simulink model "TCMSSystem"  (R2019b)
settings: configuration reference "ConfigSet_TCMSSystem_Reference" (kept outside this file)
model workspace (MAT data in the model file):
  Prm_TCMSSystem : Simulink.Parameter (value not decoded)
  SampleTime = 0.05
symbols that are objects in the model workspace (value not decoded): Prm_TCMSSystem
undefined symbols (not defined in the file): ADDIntervention, AK1Status, AK2Status, AKContactorStatus, AllDoorsClosed, AllLeftDoorsClosed, AllRightDoorsClosed, APS1Fault, APS1Isolated, APS1OutputVoltage, APS1Status, APS2Fault, APS2Isolated, APS2OutputVoltage, APS2Status, APSKAKContactor, ASCOEnd1, ASCOEnd2, ATBMode, ATCBypassMode, ATCStatusNotOK, ATOMode, ATPLowSpeedCutoutStatus, ATPMode, AuxCompressor, BatteryCurrent, BatteryIsolationContactor, BatteryTemperature, BatteryVoltage, BCG1Fault, BCG1Isolated, BCG1IsolationFailed, BCG1OutputCurrent, BCG1Status, BCG2Fault, BCG2Isolated, BCG2OutputCurrent, BCG2Status, BCGOutputVoltage, BECU1AxleLockedWheelSet1, BECU2AxleLockedWheelSet2, BECUFaulty, BECUMajorFault, BECUMinorFault, BECUStatus, BIC1Inside, BIC1Outside, BIC2Inside, BIC2Outside, Bogie, Bogie1WSPStatus, Bogie2WSPStatus, BogieFaulty, BogieIsolationStatus, BogieSupportedMass, BrakeCylinderPressureGauge, BrakeLoopCBTripped, BrakeLoopOpenTL, BrakeTrainLineStatus, BrakingDemand ... (+215)
libraries: TimersLib x257, simulink x137, LatchesLib x42, VectorOperationsLib x15, TestBenchLib x12, MathOperationsLib x2, FiltersLib x1
(part 6 of 16)

== system TCMSSystem/TCMSSystemPerVehicle/EnabledTCMSVehicle/TCMSElectrical/ElectricalDisplay/FireDetectionScreen ==
  note: FireDetectionScreen
  note: 1. RCCB Tripped
      | 2. Supply Fan Tripped
      | 3. External Smoke Detected
      | 4. Emergency Inverter Tripped
      | 5. HVAC Fire Mode
      | 6. HVAC Reduced Mode
      | 7. HVAC Group MCB Tripped
      | 8. HVAC Major Fault
  BusIn : Inport
  CommonConfig : Inport  Port=2
  In Bus Element : Inport  Port=3  PortName=ElectricalSignals  Element=HVACFaults
  In Bus Element1 : Inport  Port=3  PortName=ElectricalSignals  Element=FDUFailure
  In Bus Element3 : Inport  Port=3  PortName=ElectricalSignals  Element=SmokeAlarmCABArea
  In Bus Element4 : Inport  Port=3  PortName=ElectricalSignals  Element=HeatAlarmEDB
  In Bus Element5 : Inport  Port=3  PortName=ElectricalSignals  Element=FDUStatus
  In Bus Element6 : Inport  Port=3  PortName=ElectricalSignals  Element=SFARStatus
  In Bus Element7 : Inport  Port=3  PortName=ElectricalSignals  Element=UFARStatus
  In Bus Element2 : Inport  Port=3  PortName=ElectricalSignals  Element=InternalFireAlarmTLActive
  In Bus Element9 : Inport  Port=3  PortName=ElectricalSignals  Element=CabActive
  Bus Assignment9 : BusAssignment  AssignedSignals=UnderframeFireAlarmStatus,SaloonFireAlarmStatus,SensorFireAlarmStatus,FireDetectionUnit,InternalFire,ExternalSmoke,SmokeAlarmCABArea,HeatAlarmEDB,FDUFault,SFARFault
  Bus Selector : BusSelector  OutputSignals=HasCab
  Constant : Constant  Value=3
  Constant1 : Constant
  Data Type Conversion{,1..7} (8 alike) : DataTypeConversion
  ExternalSmoke : Selector  InputPortWidth=7  IndexOptions=Index vector (dialog)  Indices=[3]  OutputSizes=1
  FireMode : Selector  InputPortWidth=7  IndexOptions=Index vector (dialog)  Indices=[5]  OutputSizes=1
  OR : Logic  Operator=OR  Inputs=3  AllPortsSameDT=off  OutDataTypeStr=boolean
  OR1 : Logic  AllPortsSameDT=off  OutDataTypeStr=boolean
  OR2 : Logic  AllPortsSameDT=off  OutDataTypeStr=boolean
  OR3 : Logic  Operator=OR  AllPortsSameDT=off  OutDataTypeStr=boolean
  Switch : Switch  Criteria=u2 > Threshold
  BusOut : Outport
  wires:
  BusIn/1 -> Bus Assignment9/1
  Switch/1 -> Bus Assignment9/4
  Bus Assignment9/1 -> BusOut/1
  ExternalSmoke/1 -> Bus Assignment9/7
  In Bus Element/1 -> ExternalSmoke/1, FireMode/1
  OR/1 -> OR1/1, Switch/2
  In Bus Element6/1 -> Data Type Conversion3/1
  In Bus Element3/1 -> Data Type Conversion1/1
  Data Type Conversion/1 -> Bus Assignment9/9
  Data Type Conversion1/1 -> Bus Assignment9/8
  Data Type Conversion2/1 -> Bus Assignment9/5
  Data Type Conversion3/1 -> Bus Assignment9/3
  In Bus Element5/1 -> Data Type Conversion2/1
  In Bus Element1/1 -> OR2/1
  Data Type Conversion4/1 -> Bus Assignment9/10
  In Bus Element7/1 -> Data Type Conversion6/1
  In Bus Element4/1 -> OR3/1, OR/2, Data Type Conversion/1
  Data Type Conversion6/1 -> Bus Assignment9/2
  FireMode/1 -> OR/3
  In Bus Element2/1 -> OR3/2, OR/1
  In Bus Element9/1 -> OR2/2
  OR2/1 -> Data Type Conversion4/1
  Constant/1 -> Switch/1
  Constant1/1 -> Switch/3
  Data Type Conversion5/1 -> Bus Assignment9/6
  Bus Selector/1 -> OR1/2  "<HasCab>"
  OR1/1 -> Data Type Conversion5/1
  CommonConfig/1 -> Bus Selector/1
  OR3/1 -> Data Type Conversion7/1
  Data Type Conversion7/1 -> Bus Assignment9/11

== system TCMSSystem/TCMSSystemPerVehicle/EnabledTCMSVehicle/TCMSElectrical/ElectricalDisplay/FireDetectorScreen ==
  note: MiscellaneaScreen
  BusIn : Inport
  In Bus Element2 : Inport  Port=2  PortName=ElectricalSignals  Element=HeatAlarmEDB
  In Bus Element3 : Inport  Port=2  PortName=ElectricalSignals  Element=SmokeAlarmCABArea
  Bus Assignment7 : BusAssignment  AssignedSignals=HVAC1FireSmokeActive,EDBHeatAlarmActive,CABSmokeAlarmActive
  Bus Selector : BusSelector  OutputSignals=HVACFireMode
  Data Type Conversion : DataTypeConversion
  Data Type Conversion1 : DataTypeConversion
  Data Type Conversion2 : DataTypeConversion
  BusOut : Outport
  wires:
  In Bus Element2/1 -> Data Type Conversion1/1
  Bus Assignment7/1 -> BusOut/1
  BusIn/1 -> Bus Assignment7/1, Bus Selector/1
  Bus Selector/1 -> Data Type Conversion/1  "<HVACFireMode>"
  In Bus Element3/1 -> Data Type Conversion2/1
  Data Type Conversion/1 -> Bus Assignment7/2
  Data Type Conversion1/1 -> Bus Assignment7/3
  Data Type Conversion2/1 -> Bus Assignment7/4

== system TCMSSystem/TCMSSystemPerVehicle/EnabledTCMSVehicle/TCMSElectrical/ElectricalDisplay/HVACScreen ==
  note: HVACScreen
  BusIn : Inport
  In Bus Element : Inport  Port=2  PortName=ElectricalSignals  Element=HVAC1Status
  In Bus Element1 : Inport  Port=2  PortName=ElectricalSignals  Element=HVAC1SetPointTemperature
  In Bus Element2 : Inport  Port=2  PortName=ElectricalSignals  Element=HVAC1IntTemperature
  In Bus Element3 : Inport  Port=2  PortName=ElectricalSignals  Element=HVAC1ExtTemperature
  In Bus Element4 : Inport  Port=2  PortName=ElectricalSignals  Element=HVAC1Faulty
  In Bus Element5 : Inport  Port=2  PortName=ElectricalSignals  Element=HVAC1Isolated
  In Bus Element6 : Inport  Port=2  PortName=ElectricalSignals  Element=HVAC2Status
  In Bus Element7 : Inport  Port=2  PortName=ElectricalSignals  Element=HVAC2SetPointTemperature
  In Bus Element8 : Inport  Port=2  PortName=ElectricalSignals  Element=HVAC2IntTemperature
  In Bus Element9 : Inport  Port=2  PortName=ElectricalSignals  Element=HVAC2ExtTemperature
  In Bus Element10 : Inport  Port=2  PortName=ElectricalSignals  Element=HVAC2Faulty
  In Bus Element11 : Inport  Port=2  PortName=ElectricalSignals  Element=HVAC2Isolated
  In Bus Element12 : Inport  Port=2  PortName=ElectricalSignals  Element=HVACFaults
  In Bus Element13 : Inport  Port=2  PortName=ElectricalSignals  Element=MCBHVACGroupTripped
  In Bus Element16 : Inport  Port=2  PortName=ElectricalSignals  Element=NoOfAPSFailed
  In Bus Element14 : Inport  Port=3  PortName=VehicleFaults  Element=HVAC1ReducedMode
  Bus Assignment1 : BusAssignment  AssignedSignals=HVAC1Status,HVAC1SetPointTemperature,HVAC1InternalTemperature,HVAC1ExternalTemperature,HVAC1Fault,HVAC1Isolated,HVAC2Status,HVAC2SetPointTemperature,HVAC2InternalTemperature,HVAC2ExternalTemperature,HVAC2Fault,HVAC2Isolated,RCCBTripped,SupplyFanTripped,ExtSmokeDetectedinHVAC,EmergencyInverterTripped,HVACFireMode,HVACReducedMode,HVACMajorFault,HVACGroupMCBTripped,HVAC1ReducedMode,HVAC2ReducedMode
  Compare To Constant : simulink/Logic and Bit Operations/Compare To Constant  relop=>=  const=2  OutDataTypeStr=boolean
  Data Type Conversion{1..3,35..38} (7 alike) : DataTypeConversion
  Demux : Demux  Outputs=7
  Logical Operator : Logic  Operator=OR  AllPortsSameDT=off  OutDataTypeStr=boolean
  BusOut : Outport
  wires:
  Data Type Conversion38/1 -> Bus Assignment1/12
  Data Type Conversion37/1 -> Bus Assignment1/13
  In Bus Element3/1 -> Bus Assignment1/5
  In Bus Element8/1 -> Bus Assignment1/10
  In Bus Element1/1 -> Bus Assignment1/3
  Data Type Conversion36/1 -> Bus Assignment1/7
  In Bus Element6/1 -> Bus Assignment1/8
  Data Type Conversion35/1 -> Bus Assignment1/6
  Bus Assignment1/1 -> BusOut/1
  In Bus Element5/1 -> Data Type Conversion36/1
  In Bus Element2/1 -> Bus Assignment1/4
  BusIn/1 -> Bus Assignment1/1
  In Bus Element7/1 -> Bus Assignment1/9
  In Bus Element11/1 -> Data Type Conversion37/1
  In Bus Element10/1 -> Data Type Conversion38/1
  In Bus Element4/1 -> Data Type Conversion35/1
  In Bus Element9/1 -> Bus Assignment1/11
  In Bus Element/1 -> Bus Assignment1/2
  Demux/1 -> Bus Assignment1/14
  Demux/2 -> Bus Assignment1/15
  Demux/3 -> Bus Assignment1/16
  Demux/4 -> Bus Assignment1/17
  Demux/5 -> Bus Assignment1/18
  Demux/6 -> Bus Assignment1/19
  Demux/7 -> Bus Assignment1/20
  In Bus Element12/1 -> Demux/1
  In Bus Element13/1 -> Data Type Conversion1/1
  Data Type Conversion1/1 -> Bus Assignment1/21
  Data Type Conversion2/1 -> Bus Assignment1/22
  Data Type Conversion3/1 -> Bus Assignment1/23
  Compare To Constant/1 -> Data Type Conversion3/1, Logical Operator/1
  In Bus Element16/1 -> Compare To Constant/1
  Logical Operator/1 -> Data Type Conversion2/1
  In Bus Element14/1 -> Logical Operator/2

== system TCMSSystem/TCMSSystemPerVehicle/EnabledTCMSVehicle/TCMSElectrical/ElectricalDisplay/LightsScreen ==
  note: LightsScreen
  BusIn : Inport
  In Bus Element : Inport  Port=2  PortName=ElectricalSignals  Element=SaloonLightGroupStatus1
  In Bus Element1 : Inport  Port=2  PortName=ElectricalSignals  Element=SaloonLightGroupStatus2
  In Bus Element2 : Inport  Port=2  PortName=ElectricalSignals  Element=FlasherLightStatus
  Bus Assignment3 : BusAssignment  AssignedSignals=SaloonLightGroupStatus1,SaloonLightGroupStatus2,FlasherLightStatus
  Data Type Conversion32 : DataTypeConversion
  BusOut : Outport
  wires:
  Data Type Conversion32/1 -> Bus Assignment3/4
  In Bus Element1/1 -> Bus Assignment3/3
  BusIn/1 -> Bus Assignment3/1
  In Bus Element/1 -> Bus Assignment3/2
  Bus Assignment3/1 -> BusOut/1
  In Bus Element2/1 -> Data Type Conversion32/1

== system TCMSSystem/TCMSSystemPerVehicle/EnabledTCMSVehicle/TCMSElectrical/ElectricalDisplay/LowVoltageScreen ==
  note: LowVoltageScreen
  BusIn : Inport
  In Bus Element : Inport  Port=2  PortName=ElectricalSignals  Element=BatteryIsolationContactor
  In Bus Element1 : Inport  Port=2  PortName=ElectricalSignals  Element=TrainControlContactor
  Bus Assignment4 : BusAssignment  AssignedSignals=BatteryIsolationContactor,TrainControlContactor
  Data Type Conversion33 : DataTypeConversion
  Data Type Conversion34 : DataTypeConversion
  BusOut : Outport
  wires:
  Data Type Conversion33/1 -> Bus Assignment4/2
  Data Type Conversion34/1 -> Bus Assignment4/3
  In Bus Element1/1 -> Data Type Conversion34/1
  Bus Assignment4/1 -> BusOut/1
  In Bus Element/1 -> Data Type Conversion33/1
  BusIn/1 -> Bus Assignment4/1

== system TCMSSystem/TCMSSystemPerVehicle/EnabledTCMSVehicle/TCMSElectrical/ElectricalDisplay/MediumVoltageScreen ==
  note: MediumVoltageScreen
  BusIn : Inport
  In Bus Element : Inport  Port=2  PortName=ElectricalSignals  Element=MainCompressor
  In Bus Element1 : Inport  Port=2  PortName=ElectricalSignals  Element=AuxCompressor
  In Bus Element2 : Inport  Port=2  PortName=ElectricalSignals  Element=PECStatus
  Bus Assignment5 : BusAssignment  AssignedSignals=MainCompressor,AuxCompressor,PowerExtensionContactor
  Data Type Conversion23 : DataTypeConversion
  Data Type Conversion24 : DataTypeConversion
  Data Type Conversion39 : DataTypeConversion
  BusOut : Outport
  wires:
  Data Type Conversion39/1 -> Bus Assignment5/4
  Data Type Conversion23/1 -> Bus Assignment5/2
  Data Type Conversion24/1 -> Bus Assignment5/3
  Bus Assignment5/1 -> BusOut/1
  BusIn/1 -> Bus Assignment5/1
  In Bus Element/1 -> Data Type Conversion23/1
  In Bus Element1/1 -> Data Type Conversion24/1
  In Bus Element2/1 -> Data Type Conversion39/1

== system TCMSSystem/TCMSSystemPerVehicle/EnabledTCMSVehicle/TCMSElectrical/ElectricalDisplay/MiscellaneaScreen ==
  note: Changing as per customer comment.
  note: MiscellaneaScreen
  BusIn : Inport
  In Bus Element1 : Inport  Port=2  PortName=ElectricalSignals  Element=ObstacleDetected
  In Bus Element : Inport  Port=3  PortName=TractionSignals  Element=VehicleDerailed
  In Bus Element2 : Inport  Port=4  PortName=VehicleFaults  Element=ODDFailure
  Bus Assignment7 : BusAssignment  AssignedSignals=ObstructionDetectedLeft,ObstructionDetectedRight,DerailmentDetectedLeft,DerailmentDetectedRight
  Data Type Conversion : DataTypeConversion
  Data Type Conversion1 : DataTypeConversion
  Logical Operator : Logic  Operator=OR  AllPortsSameDT=off  OutDataTypeStr=boolean
  NoFaultSoFar : Constant  Value=0
  BusOut : Outport
  wires:
  BusIn/1 -> Bus Assignment7/1
  Bus Assignment7/1 -> BusOut/1
  Logical Operator/1 -> Data Type Conversion/1
  In Bus Element/1 -> Data Type Conversion1/1
  NoFaultSoFar/1 -> Bus Assignment7/4
  Data Type Conversion/1 -> Bus Assignment7/3
  Data Type Conversion1/1 -> Bus Assignment7/5
  In Bus Element1/1 -> Logical Operator/1
  In Bus Element2/1 -> Logical Operator/2, Bus Assignment7/2

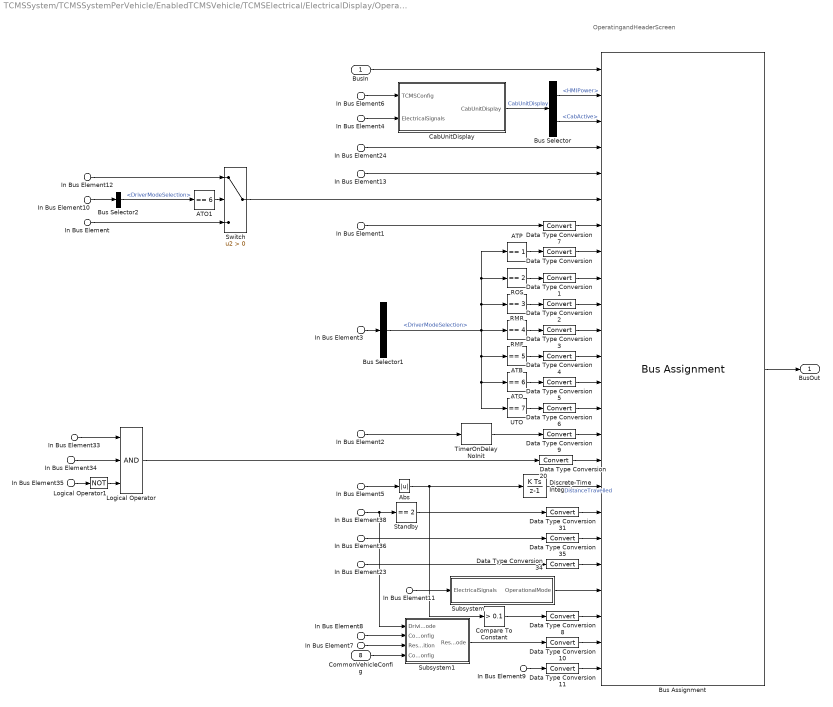
== system TCMSSystem/TCMSSystemPerVehicle/EnabledTCMSVehicle/TCMSElectrical/ElectricalDisplay/OperatingandHeaderScreen ==
  note: OperatingandHeaderScreen
  BusIn : Inport
  In Bus Element6 : Inport  Port=2  PortName=TCMSSystemVehicleConfig
  In Bus Element8 : Inport  Port=2  PortName=TCMSSystemVehicleConfig
  In Bus Element4 : Inport  Port=3  PortName=ElectricalSignals
  In Bus Element11 : Inport  Port=3  PortName=ElectricalSignals
  In Bus Element5 : Inport  Port=3  PortName=ElectricalSignals  Element=Speedometer
  In Bus Element1 : Inport  Port=3  PortName=ElectricalSignals  Element=VCBState
  In Bus Element13 : Inport  Port=3  PortName=ElectricalSignals  Element=BatteryVoltage
  In Bus Element24 : Inport  Port=3  PortName=ElectricalSignals  Element=LineVoltage
  In Bus Element33 : Inport  Port=3  PortName=ElectricalSignals  Element=VCBTripByCI
  In Bus Element36 : Inport  Port=3  PortName=ElectricalSignals  Element=MCDR
  In Bus Element23 : Inport  Port=3  PortName=ElectricalSignals  Element=VCBIsolated
  In Bus Element9 : Inport  Port=3  PortName=ElectricalSignals  Element=PowerOFFPBPressed
  In Bus Element38 : Inport  Port=4  PortName=InputControlStates  Element=ModeSelector
  In Bus Element : Inport  Port=4  PortName=InputControlStates  Element=TractionBrakeController
  In Bus Element3 : Inport  Port=5  PortName=CBTC
  In Bus Element10 : Inport  Port=5  PortName=CBTC
  In Bus Element2 : Inport  Port=5  PortName=CBTC  Element=ATCBypassState
  In Bus Element12 : Inport  Port=5  PortName=CBTC  Element=ATOTBDemandPct
  In Bus Element34 : Inport  Port=6  PortName=VehicleFaults  Element=CIFailure
  In Bus Element35 : Inport  Port=6  PortName=VehicleFaults  Element=CIIsolated
  In Bus Element7 : Inport  Port=7  PortName=CouplingSystem  Element=RescueModeCondition
  CommonVehicleConfig : Inport  Port=8
  ATB : simulink/Logic and Bit Operations/Compare To Constant  relop===  const=5  OutDataTypeStr=boolean
  ATO : simulink/Logic and Bit Operations/Compare To Constant  relop===  const=6  OutDataTypeStr=boolean
  ATO1 : simulink/Logic and Bit Operations/Compare To Constant  relop===  const=6  OutDataTypeStr=boolean
  ATP : simulink/Logic and Bit Operations/Compare To Constant  relop===  const=1  OutDataTypeStr=boolean
  Abs : Abs
  Bus Assignment : BusAssignment  AssignedSignals=HMIPower,CabActive,LineVoltage,BatteryVoltage,TBCPosition,VCBState,ATPMode,ROSMode,RMRMode,RMFMode,ATBMode,ATOMode,UTOMode,ATCBypassMode,VCBTripCommandStatus,Odometer,StandbyMode,Coupled,VCBIsolated,OperationalMode,EnableToRun,RescueMode,PowerOffPressed
  Bus Selector : BusSelector  OutputSignals=HMIPower,CabActive
  Bus Selector1 : BusSelector  OutputSignals=DriverModeSelection
  Bus Selector2 : BusSelector  OutputSignals=DriverModeSelection
  CabUnitDisplay : Subsystem
  Compare To Constant : simulink/Logic and Bit Operations/Compare To Constant  relop=>  const=0.1  OutDataTypeStr=boolean
  Data Type Conversion{,1..11,20,31,34..35} (16 alike) : DataTypeConversion
  Discrete-Time Integrator : DiscreteIntegrator  SampleTime=0.05  ICPrevOutput=DiscIntNeverNeededParam  ICPrevScaledInput=DiscIntNeverNeededParam
  Logical Operator : Logic  Inputs=3  AllPortsSameDT=off  OutDataTypeStr=boolean
  Logical Operator1 : Logic  Operator=NOT  AllPortsSameDT=off  OutDataTypeStr=boolean
  RMF : simulink/Logic and Bit Operations/Compare To Constant  relop===  const=4  OutDataTypeStr=boolean
  RMR : simulink/Logic and Bit Operations/Compare To Constant  relop===  const=3  OutDataTypeStr=boolean
  ROS : simulink/Logic and Bit Operations/Compare To Constant  relop===  const=2  OutDataTypeStr=boolean
  Standby : simulink/Logic and Bit Operations/Compare To Constant  relop===  const=2  OutDataTypeStr=boolean
  Subsystem : Subsystem
  Subsystem1 : Subsystem
  Switch : Switch  Criteria=u2 > Threshold
  TimerOnDelay NoInit : TimersLib/TimerOnDelay NoInit  UpperSaturationLimit=1.5  OutputTime=off  SampleTime=-1
      settings: SourceProductName=Sydac Utilities
  UTO : simulink/Logic and Bit Operations/Compare To Constant  relop===  const=7  OutDataTypeStr=boolean
  BusOut : Outport
  wires:
  BusIn/1 -> Bus Assignment/1
  Bus Assignment/1 -> BusOut/1
  In Bus Element33/1 -> Logical Operator/1
  In Bus Element38/1 -> Subsystem1/1(DrivingMode), Standby/1
  Standby/1 -> Data Type Conversion31/1
  In Bus Element5/1 -> Abs/1
  In Bus Element3/1 -> Bus Selector1/1
  Bus Selector1/1 -> ATP/1, ROS/1, RMR/1, RMF/1, ATB/1, ATO/1, UTO/1  "<DriverModeSelection>"
  RMF/1 -> Data Type Conversion3/1
  ATO/1 -> Data Type Conversion5/1
  UTO/1 -> Data Type Conversion6/1
  RMR/1 -> Data Type Conversion2/1
  ATP/1 -> Data Type Conversion/1
  ROS/1 -> Data Type Conversion1/1
  ATB/1 -> Data Type Conversion4/1
  In Bus Element1/1 -> Data Type Conversion7/1
  Data Type Conversion7/1 -> Bus Assignment/7
  Switch/1 -> Bus Assignment/6
  In Bus Element13/1 -> Bus Assignment/5
  In Bus Element24/1 -> Bus Assignment/4
  Bus Selector/2 -> Bus Assignment/3  "<CabActive>"
  CabUnitDisplay/1(CabUnitDisplay) -> Bus Selector/1  "CabUnitDisplay"
  Bus Selector/1 -> Bus Assignment/2  "<HMIPower>"
  In Bus Element4/1 -> CabUnitDisplay/2(ElectricalSignals)
  In Bus Element6/1 -> CabUnitDisplay/1(TCMSConfig)
  Data Type Conversion/1 -> Bus Assignment/8
  Data Type Conversion1/1 -> Bus Assignment/9
  Data Type Conversion2/1 -> Bus Assignment/10
  Data Type Conversion3/1 -> Bus Assignment/11
  Data Type Conversion4/1 -> Bus Assignment/12
  Data Type Conversion5/1 -> Bus Assignment/13
  Data Type Conversion6/1 -> Bus Assignment/14
  In Bus Element2/1 -> TimerOnDelay NoInit/1
  Data Type Conversion20/1 -> Bus Assignment/16
  Data Type Conversion31/1 -> Bus Assignment/18
  Discrete-Time Integrator/1 -> Bus Assignment/17  "DistanceTravelled"
  In Bus Element36/1 -> Data Type Conversion35/1
  In Bus Element34/1 -> Logical Operator/2
  Logical Operator1/1 -> Logical Operator/3
  In Bus Element35/1 -> Logical Operator1/1
  Logical Operator/1 -> Data Type Conversion20/1
  Data Type Conversion35/1 -> Bus Assignment/19
  Data Type Conversion34/1 -> Bus Assignment/20
  In Bus Element23/1 -> Data Type Conversion34/1
  Subsystem/1(OperationalMode) -> Bus Assignment/21
  Compare To Constant/1 -> Data Type Conversion8/1
  Abs/1 -> Compare To Constant/1, Discrete-Time Integrator/1
  Data Type Conversion8/1 -> Bus Assignment/22
  TimerOnDelay NoInit/1 -> Data Type Conversion9/1
  Data Type Conversion9/1 -> Bus Assignment/15
  In Bus Element7/1 -> Subsystem1/3(RescureModeCondition)
  Data Type Conversion10/1 -> Bus Assignment/23
  In Bus Element8/1 -> Subsystem1/2(CommonConfig)
  Subsystem1/1(RescueMode) -> Data Type Conversion10/1
  CommonVehicleConfig/1 -> Subsystem1/4(CommonVehicleConfig)
  In Bus Element9/1 -> Data Type Conversion11/1
  Data Type Conversion11/1 -> Bus Assignment/24
  In Bus Element11/1 -> Subsystem/1(ElectricalSignals)
  In Bus Element/1 -> Switch/3
  In Bus Element10/1 -> Bus Selector2/1
  Bus Selector2/1 -> ATO1/1  "<DriverModeSelection>"
  ATO1/1 -> Switch/2
  In Bus Element12/1 -> Switch/1

== system TCMSSystem/TCMSSystemPerVehicle/EnabledTCMSVehicle/TCMSElectrical/ElectricalDisplay/PantographInterlockScreen ==
  note: PantographInterlockScreen
  BusIn : Inport
  Bus Assignment6 : BusAssignment  AssignedSignals=EGSOperatedACPM,EGSOperatedOSPM
  Constant : Constant  Value=0
  BusOut : Outport
  wires:
  Constant/1 -> Bus Assignment6/2, Bus Assignment6/3
  BusIn/1 -> Bus Assignment6/1
  Bus Assignment6/1 -> BusOut/1

== system TCMSSystem/TCMSSystemPerVehicle/EnabledTCMSVehicle/TCMSElectrical/ElectricalDisplay/VCBInterlockScreen ==
  note: VCBInterlockScreen
  BusIn : Inport
  In Bus Element1 : Inport  Port=2  PortName=ElectricalSignals  Element=NoLineVoltage
  In Bus Element2 : Inport  Port=2  PortName=ElectricalSignals  Element=AK1Status
  In Bus Element3 : Inport  Port=2  PortName=ElectricalSignals  Element=K1Status
  In Bus Element4 : Inport  Port=2  PortName=ElectricalSignals  Element=AK2Status
  In Bus Element5 : Inport  Port=2  PortName=ElectricalSignals  Element=K2Status
  In Bus Element : Inport  Port=2  PortName=ElectricalSignals  Element=VCBTripByCI
  In Bus Element11 : Inport  Port=2  PortName=ElectricalSignals  Element=VCBTripByAPS
  In Bus Element12 : Inport  Port=2  PortName=ElectricalSignals  Element=VCBI_ACOvercurrent
  In Bus Element7 : Inport  Port=3  PortName=VehicleFaults  Element=VCBOpenedByACOvercurrent
  In Bus Element8 : Inport  Port=3  PortName=VehicleFaults  Element=VCBOpenedByMTrProtection
  In Bus Element9 : Inport  Port=3  PortName=VehicleFaults  Element=VCBOpenedByAPS
  In Bus Element10 : Inport  Port=3  PortName=VehicleFaults  Element=TransformerOilTemperatureTooHigh
  In Bus Element6 : Inport  Port=3  PortName=VehicleFaults  Element=APSGroup1Failure
  Bus Assignment8 : BusAssignment  AssignedSignals=TransformerOilTemperature,VCBOpenedByACOverCurrent,VCBOpenedByMTrProtection,VCBOpenedByICM,VCBOpenedByICDM,VCBOpenedByAPS,NoLineVoltage,APSKAKContactor
  Constant : Constant  Value=0
  Data Type Conversion{1..4,41..42} (6 alike) : DataTypeConversion
  OR1 : Logic  Operator=OR  AllPortsSameDT=off  OutDataTypeStr=boolean
  OR{2..5,7..8} (6 alike) : Logic  AllPortsSameDT=off  OutDataTypeStr=boolean
  OR6 : Logic  Operator=OR  AllPortsSameDT=off  OutDataTypeStr=boolean
  OR9 : Logic  Operator=OR  AllPortsSameDT=off  OutDataTypeStr=boolean
  BusOut : Outport
  wires:
  In Bus Element3/1 -> OR7/1
  In Bus Element4/1 -> OR8/2
  OR6/1 -> Data Type Conversion42/1
  In Bus Element1/1 -> Data Type Conversion41/1
  Data Type Conversion42/1 -> Bus Assignment8/9
  BusIn/1 -> Bus Assignment8/1
  In Bus Element5/1 -> OR8/1
  Data Type Conversion41/1 -> Bus Assignment8/8
  Bus Assignment8/1 -> BusOut/1
  In Bus Element2/1 -> OR7/2
  OR2/1 -> Data Type Conversion4/1
  OR3/1 -> OR9/1
  In Bus Element9/1 -> OR1/1
  OR5/1 -> Data Type Conversion1/1
  In Bus Element6/1 -> OR1/2
  Data Type Conversion1/1 -> Bus Assignment8/7
  In Bus Element11/1 -> OR5/1, OR4/1, OR3/1, OR2/1
  In Bus Element10/1 -> OR2/2
  In Bus Element7/1 -> OR3/2
  In Bus Element8/1 -> OR4/2
  OR1/1 -> OR5/2
  OR4/1 -> Data Type Conversion2/1
  Data Type Conversion2/1 -> Bus Assignment8/4
  Data Type Conversion3/1 -> Bus Assignment8/3
  Data Type Conversion4/1 -> Bus Assignment8/2
  In Bus Element/1 -> Bus Assignment8/6
  Constant/1 -> Bus Assignment8/5
  OR8/1 -> OR6/2
  OR7/1 -> OR6/1
  OR9/1 -> Data Type Conversion3/1
  In Bus Element12/1 -> OR9/2

== system TCMSSystem/TCMSSystemPerVehicle/EnabledTCMSVehicle/TCMSElectrical/ElectricalDisplay/WFLScreen ==
  note: WFLScreen
  BusIn : Inport
  In Bus Element : Inport  Port=2  PortName=ElectricalSignals  Element=WFLStatus
  In Bus Element1 : Inport  Port=2  PortName=ElectricalSignals  Element=WFLOilLevelStatus
  In Bus Element2 : Inport  Port=2  PortName=ElectricalSignals  Element=WFLPump1Status
  In Bus Element3 : Inport  Port=2  PortName=ElectricalSignals  Element=WFLPump2Status
  In Bus Element4 : Inport  Port=2  PortName=ElectricalSignals  Element=WFLFault
  In Bus Element5 : Inport  Port=2  PortName=ElectricalSignals  Element=WFLIsolated
  Bus Assignment2 : BusAssignment  AssignedSignals=WFLStatus,WFLOilLevelStatus,WFLPump1Status,WFLPump2Status,WFLFault,WFLIsolated
  BusOut : Outport
  wires:
  In Bus Element3/1 -> Bus Assignment2/5
  In Bus Element2/1 -> Bus Assignment2/4
  In Bus Element1/1 -> Bus Assignment2/3
  BusIn/1 -> Bus Assignment2/1
  Bus Assignment2/1 -> BusOut/1
  In Bus Element/1 -> Bus Assignment2/2
  In Bus Element4/1 -> Bus Assignment2/6
  In Bus Element5/1 -> Bus Assignment2/7

== system TCMSSystem/TCMSSystemPerVehicle/EnabledTCMSVehicle/TCMSPantograph/PantographDisplay/CabUnitDisplay ==
  TCMSConfig : Inport
  ElectricalSignals : Inport  Port=2
  AND : Logic  AllPortsSameDT=off  OutDataTypeStr=boolean
  Bus Selector : BusSelector  OutputSignals=CabActive
  Bus Selector1 : BusSelector  OutputSignals=HasCab
  CabActiveUnitDisplay : Subsystem  TreatAsAtomicUnit=on
  CabInActiveUnitDisplay : Subsystem  TreatAsAtomicUnit=on
  Data Type Conversion : DataTypeConversion  OutDataTypeStr=uint32
  If : If
  Merge : Merge
  CabUnitDisplay : Outport
  wires:
  ElectricalSignals/1 -> CabActiveUnitDisplay/1(ElectricalSignals), Bus Selector/1
  TCMSConfig/1 -> Bus Selector1/1
  Bus Selector1/1 -> AND/1  "<HasCab>"
  Bus Selector/1 -> AND/2  "<CabActive>"
  AND/1 -> Data Type Conversion/1
  Data Type Conversion/1 -> If/1
  If/1 -> CabActiveUnitDisplay/Action
  If/2 -> CabInActiveUnitDisplay/Action
  CabActiveUnitDisplay/1(Out1) -> Merge/1
  CabInActiveUnitDisplay/1(Out1) -> Merge/2
  Merge/1 -> CabUnitDisplay/1

== system TCMSSystem/TCMSSystemPerVehicle/EnabledTCMSVehicle/TCMSPantograph/PantographDisplay/TCMSVehicleInfo ==
  In Bus Element3 : Inport  PortName=PantographSystem  Element=PantoUpStatus
  In Bus Element4 : Inport  PortName=PantographSystem  Element=PantoDownStatus
  In Bus Element5 : Inport  PortName=PantographSystem  Element=PantoIsolatedStatus
  In Bus Element6 : Inport  PortName=PantographSystem  Element=PantoRising
  In Bus Element7 : Inport  PortName=PantographSystem  Element=PantoLowering
  In Bus Element : Inport  PortName=PantographSystem  Element=PantographPosition
  In Bus Element1 : Inport  PortName=PantographSystem  Element=PantographFault
  In Bus Element2 : Inport  PortName=PantographSystem  Element=PantoADDFaultMessage
  In Bus Element8 : Inport  PortName=PantographSystem  Element=PantoORDFaultMessage
  In Bus Element9 : Inport  PortName=PantographSystem  Element=PantoRaiseFailureMessage
  Bus Creator : BusCreator  Inputs=10
  Data Type Conversion{,1..8} (9 alike) : DataTypeConversion  OutDataTypeStr=double
  TCMSVehicleInfo : Outport
  wires:
  Bus Creator/1 -> TCMSVehicleInfo/1
  In Bus Element7/1 -> Data Type Conversion/1
  In Bus Element6/1 -> Data Type Conversion1/1
  In Bus Element5/1 -> Data Type Conversion2/1
  In Bus Element3/1 -> Data Type Conversion4/1
  In Bus Element4/1 -> Data Type Conversion3/1
  Data Type Conversion/1 -> Bus Creator/6  "VehiclePantoLowering"
  Data Type Conversion1/1 -> Bus Creator/5  "VehiclePantoRising"
  Data Type Conversion2/1 -> Bus Creator/4  "VehiclePantoIsolated"
  Data Type Conversion3/1 -> Bus Creator/3  "VehiclePantoDown"
  Data Type Conversion4/1 -> Bus Creator/2  "VehiclePantoUp"
  In Bus Element/1 -> Bus Creator/1  "PantographPosition"
  In Bus Element1/1 -> Data Type Conversion5/1
  In Bus Element2/1 -> Data Type Conversion6/1
  In Bus Element8/1 -> Data Type Conversion7/1
  Data Type Conversion5/1 -> Bus Creator/7  "PantographFault"
  Data Type Conversion6/1 -> Bus Creator/8  "PantoADDFaultMessage"
  Data Type Conversion7/1 -> Bus Creator/9  "PantoORDFaultMessage"
  In Bus Element9/1 -> Data Type Conversion8/1
  Data Type Conversion8/1 -> Bus Creator/10  "PantoRaiseFailureMessage"

== system TCMSSystem/TCMSSystemPerVehicle/EnabledTCMSVehicle/TCMSPneumatics/PneumaticsDisplay/CabUnitDisplay ==
  TCMSConfig : Inport
  ElectricalSignals : Inport  Port=2
  AND : Logic  AllPortsSameDT=off  OutDataTypeStr=boolean
  Bus Selector : BusSelector  OutputSignals=CabActive
  Bus Selector1 : BusSelector  OutputSignals=HasCab
  CabActiveUnitDisplay : Subsystem  TreatAsAtomicUnit=on
  CabInActiveUnitDisplay : Subsystem  TreatAsAtomicUnit=on
  Data Type Conversion : DataTypeConversion  OutDataTypeStr=uint32
  If : If
  Merge : Merge
  CabUnitDisplay : Outport
  wires:
  Merge/1 -> CabUnitDisplay/1
  CabInActiveUnitDisplay/1(Out1) -> Merge/2
  CabActiveUnitDisplay/1(Out1) -> Merge/1
  If/2 -> CabInActiveUnitDisplay/Action
  If/1 -> CabActiveUnitDisplay/Action
  Data Type Conversion/1 -> If/1
  AND/1 -> Data Type Conversion/1
  Bus Selector/1 -> AND/2  "<CabActive>"
  Bus Selector1/1 -> AND/1  "<HasCab>"
  TCMSConfig/1 -> Bus Selector1/1
  ElectricalSignals/1 -> Bus Selector/1, CabActiveUnitDisplay/1(ElectricalSignals)

== system TCMSSystem/TCMSSystemPerVehicle/EnabledTCMSVehicle/TCMSPneumatics/PneumaticsDisplay/For Each Subsystem ==
  Bogie : Inport  Partition=on  PartitionDimension=1  PartitionWidth=1  PartitionOffset=0
  Bus Assignment : BusAssignment  AssignedSignals=BrakeCylinderPressureGauge,ParkBrakePressureGauge
  Bus Selector : BusSelector  OutputSignals=ServiceBrakeSwitchStatus,PrakingBrakeSwitchStatus,AirSuspensionPressure
  Bus Selector5 : BusSelector  OutputSignals=BrakeCylinderPressureGauge,ParkBrakePressureGauge
  Constant : Constant  Value=0  OutDataTypeStr=Bus: BD_TCMSSystem_Out_Vehicle_Display_PneumaticsSystem_Bogie
  For Each : ForEach  DisableCoverage=on
  BogieGauge : Outport  ConcatenationDimension=1
  BrakeCylinderPressureGauge : Outport  Port=2  ConcatenationDimension=1
  ServiceBrakeSwitchStatus : Outport  Port=3  ConcatenationDimension=1
  ParkingBrakeSwitchStatus : Outport  Port=4  ConcatenationDimension=1
  AirSuspensionPressure : Outport  Port=5  ConcatenationDimension=1
  wires:
  Bogie/1 -> Bus Selector/1, Bus Selector5/1
  Bus Selector/1 -> ServiceBrakeSwitchStatus/1  "<ServiceBrakeSwitchStatus>"
  Bus Selector/2 -> ParkingBrakeSwitchStatus/1  "<PrakingBrakeSwitchStatus>"
  Bus Selector/3 -> AirSuspensionPressure/1  "<AirSuspensionPressure>"
  Bus Selector5/1 -> Bus Assignment/2, BrakeCylinderPressureGauge/1  "<BrakeCylinderPressureGauge>"
  Bus Selector5/2 -> Bus Assignment/3  "<ParkBrakePressureGauge>"
  Constant/1 -> Bus Assignment/1
  Bus Assignment/1 -> BogieGauge/1

== system TCMSSystem/TCMSSystemPerVehicle/EnabledTCMSVehicle/TCMSPneumatics/PneumaticsDisplay/For Each Subsystem1 ==
  Bogie : Inport  Partition=on  PartitionDimension=1  PartitionWidth=1  PartitionOffset=0
  Bus Selector5 : BusSelector  OutputSignals=BECU1EmergencyBrakeFailure,BECU2EmergencyBrakeFailure,BECU1ServiceBrakeFailure,BECU1BrakeNotApplied,BECU1BrakeNotReleased,BECU1CarLoadPressureLow,BECU2CarLoadPressureLow,BECULowRPressure,AirSuspensionBogie1Deflated,BECU1LoadPressureLow
  For Each : ForEach  DisableCoverage=on
  BECU1EmergencyBrakeFailure : Outport  ConcatenationDimension=1
  BECU2EmergencyBrakeFailure : Outport  Port=2  ConcatenationDimension=1
  BECU1ServiceBrakeFailure : Outport  Port=3  ConcatenationDimension=1
  BECU1BrakeNotApplied : Outport  Port=4  ConcatenationDimension=1
  BECU1BrakeNotReleased : Outport  Port=5  ConcatenationDimension=1
  BECU1CarLoadPressureLow : Outport  Port=6  ConcatenationDimension=1
  BECU2CarLoadPressureLow : Outport  Port=7  ConcatenationDimension=1
  BECULowRPressure : Outport  Port=8  ConcatenationDimension=1
  ASBogie1Deflated : Outport  Port=9  ConcatenationDimension=1
  BECU1LoadPressureLow : Outport  Port=10  ConcatenationDimension=1
  wires:
  Bogie/1 -> Bus Selector5/1
  Bus Selector5/4 -> BECU1BrakeNotApplied/1  "<BECU1BrakeNotApplied>"
  Bus Selector5/1 -> BECU1EmergencyBrakeFailure/1  "<BECU1EmergencyBrakeFailure>"
  Bus Selector5/3 -> BECU1ServiceBrakeFailure/1  "<BECU1ServiceBrakeFailure>"
  Bus Selector5/5 -> BECU1BrakeNotReleased/1  "<BECU1BrakeNotReleased>"
  Bus Selector5/2 -> BECU2EmergencyBrakeFailure/1  "<BECU2EmergencyBrakeFailure>"
  Bus Selector5/8 -> BECULowRPressure/1  "<BECULowRPressure>"
  Bus Selector5/6 -> BECU1CarLoadPressureLow/1  "<BECU1CarLoadPressureLow>"
  Bus Selector5/7 -> BECU2CarLoadPressureLow/1  "<BECU2CarLoadPressureLow>"
  Bus Selector5/10 -> BECU1LoadPressureLow/1  "<BECU1LoadPressureLow>"
  Bus Selector5/9 -> ASBogie1Deflated/1  "<AirSuspensionBogie1Deflated>"

== system TCMSSystem/TCMSSystemPerVehicle/EnabledTCMSVehicle/TCMSPneumatics/PneumaticsDisplay/Subsystem ==
  InP : Inport
  Speed : Inport  Port=2
  ED : Inport  Port=3
  IsT? : Inport  Port=4
  Abs : Abs
  Compare To Constant1 : simulink/Logic and Bit Operations/Compare To Constant  relop=>=  const=1.75  OutDataTypeStr=boolean
  Compare To Constant2 : simulink/Logic and Bit Operations/Compare To Constant  relop=>  const=1  OutDataTypeStr=boolean
  Constant : Constant  Value=0
  Logical Operator12 : Logic  Inputs=3  AllPortsSameDT=off  OutDataTypeStr=boolean
  Switch1 : Switch  Criteria=u2 > Threshold  Threshold=1.75
  OutP : Outport
  wires:
  Logical Operator12/1 -> Switch1/2
  IsT?/1 -> Logical Operator12/3
  Switch1/1 -> OutP/1
  ED/1 -> Compare To Constant2/1
  Constant/1 -> Switch1/1
  Compare To Constant1/1 -> Logical Operator12/1
  Abs/1 -> Compare To Constant1/1
  Speed/1 -> Abs/1
  InP/1 -> Switch1/3
  Compare To Constant2/1 -> Logical Operator12/2

== system TCMSSystem/TCMSSystemPerVehicle/EnabledTCMSVehicle/TCMSPneumatics/PneumaticsDisplay/Subsystem1 ==
  Fault : Inport
  Cmd : Inport  Port=2
  Data Type Conversion : DataTypeConversion
  Detect Decrease : simulink/Logic and Bit Operations/Detect Decrease  vinit=0.0  OutDataTypeStr=boolean
  Detect Increase : simulink/Logic and Bit Operations/Detect Increase  vinit=0.0  OutDataTypeStr=boolean
  Logical Operator1 : Logic  AllPortsSameDT=off  OutDataTypeStr=boolean
  SR Latch - Reset Priority : LatchesLib/SR Latch - Reset Priority  initial_condition=0
      settings: SourceProductName=Latches
  Trig : Outport
  wires:
  Data Type Conversion/1 -> Trig/1
  Detect Decrease/1 -> SR Latch - Reset Priority/2
  SR Latch - Reset Priority/1 -> Data Type Conversion/1
  Logical Operator1/1 -> SR Latch - Reset Priority/1
  Fault/1 -> Logical Operator1/1, Detect Decrease/1
  Cmd/1 -> Detect Increase/1
  Detect Increase/1 -> Logical Operator1/2

== system TCMSSystem/TCMSSystemPerVehicle/EnabledTCMSVehicle/TCMSPneumatics/PneumaticsDisplay/Subsystem2 ==
  InP : Inport
  Speed : Inport  Port=2
  ED : Inport  Port=3
  IsT? : Inport  Port=4
  Abs : Abs
  Compare To Constant1 : simulink/Logic and Bit Operations/Compare To Constant  relop=>=  const=1.75  OutDataTypeStr=boolean
  Compare To Constant2 : simulink/Logic and Bit Operations/Compare To Constant  relop=>  const=1  OutDataTypeStr=boolean
  Constant : Constant  Value=0
  Logical Operator12 : Logic  Inputs=3  AllPortsSameDT=off  OutDataTypeStr=boolean
  Switch1 : Switch  Criteria=u2 > Threshold  Threshold=1.75
  OutP : Outport
  wires:
  Compare To Constant2/1 -> Logical Operator12/2
  InP/1 -> Switch1/3
  Speed/1 -> Abs/1
  Abs/1 -> Compare To Constant1/1
  Compare To Constant1/1 -> Logical Operator12/1
  Constant/1 -> Switch1/1
  ED/1 -> Compare To Constant2/1
  Switch1/1 -> OutP/1
  IsT?/1 -> Logical Operator12/3
  Logical Operator12/1 -> Switch1/2

== system TCMSSystem/TCMSSystemPerVehicle/EnabledTCMSVehicle/TCMSPneumatics/PneumaticsDisplay/Subsystem3 ==
  Fault : Inport
  Cmd : Inport  Port=2
  Data Type Conversion : DataTypeConversion
  Detect Decrease : simulink/Logic and Bit Operations/Detect Decrease  vinit=0.0  OutDataTypeStr=boolean
  Detect Increase : simulink/Logic and Bit Operations/Detect Increase  vinit=0.0  OutDataTypeStr=boolean
  Logical Operator1 : Logic  AllPortsSameDT=off  OutDataTypeStr=boolean
  SR Latch - Reset Priority : LatchesLib/SR Latch - Reset Priority  initial_condition=0
      settings: SourceProductName=Latches
  Trig : Outport
  wires:
  Cmd/1 -> Detect Increase/1
  Fault/1 -> Detect Decrease/1, Logical Operator1/1
  Logical Operator1/1 -> SR Latch - Reset Priority/1
  SR Latch - Reset Priority/1 -> Data Type Conversion/1
  Detect Decrease/1 -> SR Latch - Reset Priority/2
  Data Type Conversion/1 -> Trig/1
  Detect Increase/1 -> Logical Operator1/2

== system TCMSSystem/TCMSSystemPerVehicle/EnabledTCMSVehicle/TCMSTractionBraking/HoldingBrakeFB_ASDeflatedExtract/For Each Subsystem ==
  Bogie : Inport  Partition=on  PartitionDimension=1  PartitionWidth=1  PartitionOffset=0
  Bus Selector5 : BusSelector  OutputSignals=BrakeCylinderPressureGauge,AirSuspensionBogie1Deflated
  For Each : ForEach  DisableCoverage=on
  BogieGauge : Outport  ConcatenationDimension=1
  Out2 : Outport  Port=2  ConcatenationDimension=1
  wires:
  Bogie/1 -> Bus Selector5/1
  Bus Selector5/1 -> BogieGauge/1  "<BrakeCylinderPressureGauge>"
  Bus Selector5/2 -> Out2/1  "<AirSuspensionBogie1Deflated>"

== system TCMSSystem/TCMSSystemPerVehicle/EnabledTCMSVehicle/TCMSTractionBraking/TractionBrakingControl/CabControlsExtract ==
  note: Added as per BEML requirement.
  note: HTE
  TCMSConfig : Inport
  In Bus Element3 : Inport  Port=2  PortName=ElectricalSignals
  In Bus Element4 : Inport  Port=3  PortName=CBTCSignals
  In Bus Element10 : Inport  Port=3  PortName=CBTCSignals  Element=RollbackDetected
  In Bus Element5 : Inport  Port=4  PortName=InputControlStates
  In Bus Element8 : Inport  Port=5  PortName=PneumaticTrainSum
  In Bus Element6 : Inport  Port=6  PortName=TractionCmd
  In Bus Element9 : Inport  Port=7  PortName=TractionBrakingBogieData
  In Bus Element2 : Inport  Port=8  PortName=DisplayControl
  In Bus Element24 : Inport  Port=8  PortName=DisplayControl  Element=ActivateHTE
  In Bus Element11 : Inport  Port=8  PortName=DisplayControl  Element=ATPLowModeActivated
  In Bus Element12 : Inport  Port=8  PortName=DisplayControl  Element=ShuntModeActivated
  In Bus Element : Inport  Port=9  PortName=Faults
  In Bus Element1 : Inport  Port=9  PortName=Faults  Element=HighTractiveEffortRequired
  In Bus Element7 : Inport  Port=10  PortName=PneumaticsSystem
  In Bus Element13 : Inport  Port=11  PortName=DynamicsIn
  AND : Logic  AllPortsSameDT=off  OutDataTypeStr=boolean
  AND1 : Logic  Operator=OR  AllPortsSameDT=off  OutDataTypeStr=boolean
  Bus Selector : BusSelector  OutputSignals=CabActive
  Bus Selector1 : BusSelector  OutputSignals=HasCab
  CabActiveTrainControl : Subsystem  TreatAsAtomicUnit=on
  CabInactiveNoTrainControl : Subsystem  TreatAsAtomicUnit=on
  Data Type Conversion : DataTypeConversion  OutDataTypeStr=uint32
  Data Type Conversion1 : DataTypeConversion
  Data Type Conversion2 : DataTypeConversion
  Detect Increase : simulink/Logic and Bit Operations/Detect Increase  vinit=0.0  OutDataTypeStr=boolean
  If : If
  Merge : Merge
  SR Latch - Reset Priority : LatchesLib/SR Latch - Reset Priority  initial_condition=0
      settings: SourceProductName=Latches
  Speed Limit Protection : Subsystem
  TractionBrakingRefCalc : Subsystem
  TractionBrakingTrainWireSource : Outport
  wires:
  Bus Selector/1 -> AND/2  "<CabActive>"
  AND/1 -> Data Type Conversion/1
  If/2 -> CabInactiveNoTrainControl/Action
  Bus Selector1/1 -> AND/1  "<HasCab>"
  In Bus Element3/1 -> Bus Selector/1, Speed Limit Protection/1(ElectricalIn)
  TCMSConfig/1 -> Bus Selector1/1
  In Bus Element2/1 -> Speed Limit Protection/4(DisplayControl), CabActiveTrainControl/1(DisplayControl)
  If/1 -> CabActiveTrainControl/Action
  Merge/1 -> TractionBrakingTrainWireSource/1  "TractionBrakingTrainWireSource"
  Data Type Conversion/1 -> If/1
  CabInactiveNoTrainControl/1(Out1) -> Merge/2
  CabActiveTrainControl/1(Out1) -> Merge/1
  In Bus Element5/1 -> Speed Limit Protection/3(IOControls), TractionBrakingRefCalc/3(InputState)
  TractionBrakingRefCalc/1(TractionCommand) -> CabActiveTrainControl/2(TractionCommand)
  TractionBrakingRefCalc/2(BrakingCommand) -> CabActiveTrainControl/3(BrakingCommand)
  In Bus Element4/1 -> Speed Limit Protection/2(CBTCIn), TractionBrakingRefCalc/2(CBTCSignals)
  TractionBrakingRefCalc/3(HoldingBrakesStatus) -> CabActiveTrainControl/4(HoldingBrakeStatus)
  Speed Limit Protection/2(TCMSSpeedLimit) -> CabActiveTrainControl/5(TCMSSpeedLimit)
  Speed Limit Protection/3(LimitActive) -> CabActiveTrainControl/6(LimitActive)
  In Bus Element6/1 -> TractionBrakingRefCalc/4(TractionCmd)
  In Bus Element8/1 -> Speed Limit Protection/6(PneumaticsTrainSum)
  In Bus Element/1 -> TractionBrakingRefCalc/5(Faults)
  In Bus Element9/1 -> Speed Limit Protection/7(TractionBrakingBogieData)
  In Bus Element24/1 -> SR Latch - Reset Priority/2
  Detect Increase/1 -> SR Latch - Reset Priority/1
  In Bus Element1/1 -> AND1/1
  SR Latch - Reset Priority/1 -> Data Type Conversion1/1
  Speed Limit Protection/4(WashModeActive) -> Data Type Conversion2/1
  Data Type Conversion1/1 -> CabActiveTrainControl/7(HTERequired)
  Data Type Conversion2/1 -> CabActiveTrainControl/8(WashModeActive)
  In Bus Element7/1 -> Speed Limit Protection/5(PneumaticsSystem)
  Speed Limit Protection/1(SpecialModesOverspeed) -> TractionBrakingRefCalc/6(SpecialModesOverspeed)
  In Bus Element10/1 -> AND1/2
  AND1/1 -> Detect Increase/1
  In Bus Element11/1 -> CabActiveTrainControl/10(ATPLowSpeedCutoutModeActive)
  In Bus Element12/1 -> CabActiveTrainControl/9(ShuntModeActive)
  In Bus Element13/1 -> TractionBrakingRefCalc/1(DynamicsIn)

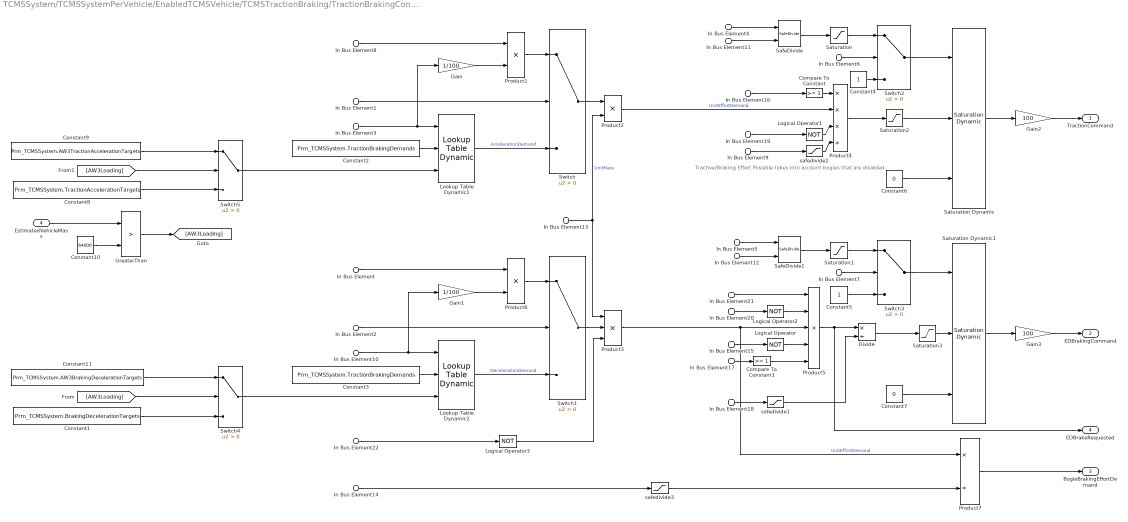
== system TCMSSystem/TCMSSystemPerVehicle/EnabledTCMSVehicle/TCMSTractionBraking/TractionBrakingControl/CentralUnitControl ==
  note: Tractive/Braking Effort Possible takes into account bogies that are disabled.
  In Bus Element6 : Inport  PortName=TractionTrainControl  Element=EnableTractionPowerLimit
  In Bus Element5 : Inport  PortName=TractionTrainControl  Element=EDBrakingPowerLimit
  In Bus Element7 : Inport  PortName=TractionTrainControl  Element=EnableEDBrakingPowerLimit
  In Bus Element8 : Inport  PortName=TractionTrainControl  Element=MaxTractionAccelerationTargetOverride
  In Bus Element : Inport  PortName=TractionTrainControl  Element=MaxBrakingDecelerationTargetOverride
  In Bus Element1 : Inport  PortName=TractionTrainControl  Element=EnableTractionTargetOverride
  In Bus Element2 : Inport  PortName=TractionTrainControl  Element=EnableBrakingTargetOverride
  In Bus Element4 : Inport  PortName=TractionTrainControl  Element=TractionPowerLimit
  In Bus Element3 : Inport  PortName=TractionTrainControl  Element=TractionCommand
  In Bus Element10 : Inport  PortName=TractionTrainControl  Element=BrakingCommand
  In Bus Element15 : Inport  PortName=TractionTrainControl  Element=HoldingBrakeStatus
  In Bus Element19 : Inport  PortName=TractionTrainControl  Element=Overspeed
  In Bus Element11 : Inport  Port=2  PortName=TractionUnitData  Element=TractivePowerPossible
  In Bus Element12 : Inport  Port=2  PortName=TractionUnitData  Element=EDBrakingPowerPossible
  In Bus Element13 : Inport  Port=2  PortName=TractionUnitData  Element=EstimatedMass
  In Bus Element16 : Inport  Port=2  PortName=TractionUnitData  Element=TractionBogiesAvailable
  In Bus Element17 : Inport  Port=2  PortName=TractionUnitData  Element=EDBrakingBogiesAvailable
  In Bus Element9 : Inport  Port=2  PortName=TractionUnitData  Element=TractiveEffortPossible
  In Bus Element18 : Inport  Port=2  PortName=TractionUnitData  Element=EDBrakingEffortPossible
  In Bus Element14 : Inport  Port=2  PortName=TractionUnitData  Element=BrakingBogiesEquipped
  In Bus Element21 : Inport  Port=3  PortName=ElectricalIn  Element=NoEB
  In Bus Element20 : Inport  Port=3  PortName=ElectricalIn  Element=LimpHomeMode
  EstimatedVehicleMass : Inport  Port=4
  In Bus Element22 : Inport  Port=5  PortName=PneumaticsSystem  Element=BrakeDemandSignalFailure
  Compare To Constant : simulink/Logic and Bit Operations/Compare To Constant  relop=>=  const=1  OutDataTypeStr=boolean
  Compare To Constant1 : simulink/Logic and Bit Operations/Compare To Constant  relop=>=  const=1  OutDataTypeStr=boolean
  Constant1 : Constant  Value=Prm_TCMSSystem.BrakingDecelerationTargets
  Constant10 : Constant  Value=64000
  Constant11 : Constant  Value=Prm_TCMSSystem.AW3BrakingDecelerationTargets
  Constant2 : Constant  Value=Prm_TCMSSystem.TractionBrakingDemands
  Constant3 : Constant  Value=Prm_TCMSSystem.TractionBrakingDemands
  Constant4 : Constant
  Constant5 : Constant
  Constant6 : Constant  Value=0
  Constant7 : Constant  Value=0
  Constant8 : Constant  Value=Prm_TCMSSystem.TractionAccelerationTargets
  Constant9 : Constant  Value=Prm_TCMSSystem.AW3TractionAccelerationTargets
  Divide : Product  Inputs=*/
  Gain : Gain  Gain=1/100
  Gain1 : Gain  Gain=1/100
  Gain2 : Gain  Gain=100
  Gain3 : Gain  Gain=100
  GreaterThan : RelationalOperator  Operator=>  OutDataTypeStr=boolean  RndMeth=Simplest
  Logical Operator{,1..3} (4 alike) : Logic  Operator=NOT  AllPortsSameDT=off  OutDataTypeStr=boolean
  Lookup Table Dynamic1 : simulink/Lookup Tables/Lookup Table Dynamic  LookUpMeth=Interpolation-Use End Values  OutDataType=fixdt('double')  OutScaling=[]  OutputDataTypeScalingMode=Specify via dialog  OutDataTypeStr=double  DoSatur=off
      settings: SourceProductName=Simulink
  Lookup Table Dynamic2 : simulink/Lookup Tables/Lookup Table Dynamic  LookUpMeth=Interpolation-Use End Values  OutDataType=fixdt('double')  OutScaling=[]  OutputDataTypeScalingMode=Specify via dialog  OutDataTypeStr=double  DoSatur=off
      settings: SourceProductName=Simulink
  Product1 : Product  Inputs=**
  Product2 : Product
  Product3 : Product  Inputs=3
  Product4 : Product  Inputs=***/
  Product5 : Product  Inputs=*****
  Product6 : Product  Inputs=**
  Product7 : Product  Inputs=*/
  SafeDivide : MathOperationsLib/SafeDivide
      settings: SourceProductName=Math Operations
  SafeDivide1 : MathOperationsLib/SafeDivide
      settings: SourceProductName=Math Operations
  Saturation{,1..3} (4 alike) : Saturate  UpperLimit=1  LowerLimit=0
  Saturation Dynamic : simulink/Discontinuities/Saturation Dynamic  OutMin=[]  OutMax=[]  OutDataTypeStr=Inherit: Same as second input  OutDataType=fixdt(1, 16)  OutScaling=2^-10  DoSatur=off
  Saturation Dynamic1 : simulink/Discontinuities/Saturation Dynamic  OutMin=[]  OutMax=[]  OutDataTypeStr=Inherit: Same as second input  OutDataType=fixdt(1, 16)  OutScaling=2^-10  DoSatur=off
  Switch{,1..5} (6 alike) : Switch  Criteria=u2 > Threshold
  safedivide1 : Saturate  UpperLimit=1e8  LowerLimit=eps
  safedivide2 : Saturate  UpperLimit=1e8  LowerLimit=eps
  safedivide3 : Saturate  UpperLimit=1e8  LowerLimit=eps
  TractionCommand : Outport
  EDBrakingCommand : Outport  Port=2
  BogieBrakingEffortDemand : Outport  Port=3
  EDBrakeRequested : Outport  Port=4
  wires:
  In Bus Element11/1 -> SafeDivide/2
  In Bus Element4/1 -> SafeDivide/1
  SafeDivide/1 -> Saturation/1
  SafeDivide1/1 -> Saturation1/1
  In Bus Element5/1 -> SafeDivide1/1
  In Bus Element12/1 -> SafeDivide1/2
  In Bus Element10/1 -> Gain1/1, Lookup Table Dynamic2/1
  In Bus Element3/1 -> Gain/1, Lookup Table Dynamic1/1
  Constant2/1 -> Lookup Table Dynamic1/2
  Switch5/1 -> Lookup Table Dynamic1/3
  Constant3/1 -> Lookup Table Dynamic2/2
  In Bus Element2/1 -> Switch1/2
  Lookup Table Dynamic2/1 -> Switch1/3  "DecelerationDemand"
  In Bus Element1/1 -> Switch/2
  Lookup Table Dynamic1/1 -> Switch/3  "AccelerationDemand"
  Gain/1 -> Product1/2
  In Bus Element8/1 -> Product1/1
  Product1/1 -> Switch/1
  Product6/1 -> Switch1/1
  Gain1/1 -> Product6/2
  In Bus Element/1 -> Product6/1
  In Bus Element13/1 -> Product2/2, Product3/1  "UnitMass"
  Switch1/1 -> Product3/2
  Switch/1 -> Product2/1
  In Bus Element9/1 -> safedivide2/1
  Product3/1 -> Product7/1, Product5/3  "UnitEffortDemand"
  Product4/1 -> Saturation2/1
  In Bus Element18/1 -> safedivide1/1
  Saturation/1 -> Switch2/1
  In Bus Element6/1 -> Switch2/2
  Constant4/1 -> Switch2/3
  In Bus Element16/1 -> Compare To Constant/1
  In Bus Element17/1 -> Compare To Constant1/1
  Saturation3/1 -> Saturation Dynamic1/2
  Saturation1/1 -> Switch3/1
  In Bus Element7/1 -> Switch3/2
  Constant5/1 -> Switch3/3
  Switch2/1 -> Saturation Dynamic/1
  Saturation2/1 -> Saturation Dynamic/2
  Switch3/1 -> Saturation Dynamic1/1
  Constant6/1 -> Saturation Dynamic/3
  Constant7/1 -> Saturation Dynamic1/3
  Saturation Dynamic1/1 -> Gain3/1
  Saturation Dynamic/1 -> Gain2/1
  Gain2/1 -> TractionCommand/1
  Gain3/1 -> EDBrakingCommand/1
  In Bus Element14/1 -> safedivide3/1
  Product7/1 -> BogieBrakingEffortDemand/1
  safedivide2/1 -> Product4/4
  safedivide3/1 -> Product7/2
  In Bus Element15/1 -> Logical Operator/1
  Logical Operator/1 -> Product5/4
  In Bus Element19/1 -> Logical Operator1/1
  Logical Operator1/1 -> Product4/3
  In Bus Element21/1 -> Product5/1
  Product5/1 -> EDBrakeRequested/1, Divide/1
  Divide/1 -> Saturation3/1
  safedivide1/1 -> Divide/2
  Logical Operator2/1 -> Product5/2
  In Bus Element20/1 -> Logical Operator2/1
  Constant10/1 -> GreaterThan/2
  Constant9/1 -> Switch5/1
  EstimatedVehicleMass/1 -> GreaterThan/1
  Constant8/1 -> Switch5/3
  GreaterThan/1 -> [AW3Loading]
  [AW3Loading] -> Switch5/2
  Constant1/1 -> Switch4/3
  Constant11/1 -> Switch4/1
  [AW3Loading] -> Switch4/2
  Switch4/1 -> Lookup Table Dynamic2/3
  Compare To Constant/1 -> Product4/1
  Compare To Constant1/1 -> Product5/5
  In Bus Element22/1 -> Logical Operator3/1
  Logical Operator3/1 -> Product3/3
  Product2/1 -> Product4/2  "UnitEffortDemand"
